simulink model "FirstAttributes"  (Simulink 7.4)
settings: Solver=ode45  StartTime=0.0  StopTime=10.0  RelTol=1e-3
settings Model: Creator=dread  LastModifiedBy=dread

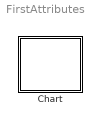
== system FirstAttributes ==
  Chart : Stateflow chart

== stateflow chart Chart ==
  state Top
    state Mid
      state In1
      state In2
      In1 -> In2
  data: data constant double
  events: event local EITHER_EDGE_EVENT
